simulink subsystem "switch_states"  (R2024a)
settings: Solver=VariableStepAuto  StartTime=0.0  StopTime=10.0  RelTol=1e-3
settings Model: Creator=javeed  LastModifiedBy=javeed

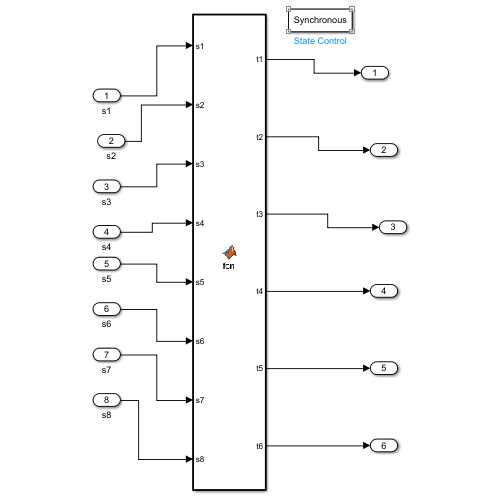
[thumbnail: Simulink's stored preview of the top-level diagram]
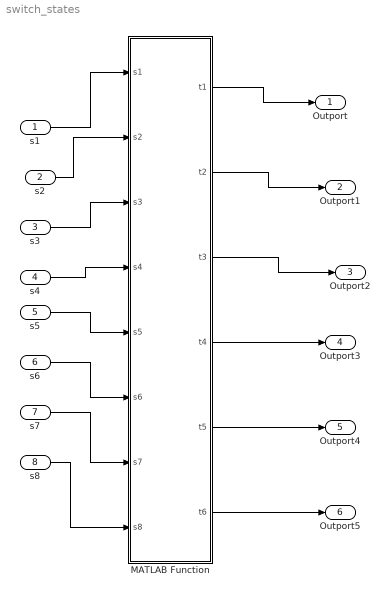
== system switch_states ==
  s1 : Inport
  s2 : Inport  Port=2
  s3 : Inport  Port=3
  s4 : Inport  Port=4
  s5 : Inport  Port=5
  s6 : Inport  Port=6
  s7 : Inport  Port=7
  s8 : Inport  Port=8
  MATLAB Function : MATLAB Function  TreatAsAtomicUnit=on
  Outport : Outport
  Outport1 : Outport  Port=2
  Outport2 : Outport  Port=3
  Outport3 : Outport  Port=4
  Outport4 : Outport  Port=5
  Outport5 : Outport  Port=6
  wires:
  s1/1 -> MATLAB Function/1(s1)
  s2/1 -> MATLAB Function/2(s2)
  s3/1 -> MATLAB Function/3(s3)
  s4/1 -> MATLAB Function/4(s4)
  s5/1 -> MATLAB Function/5(s5)
  s6/1 -> MATLAB Function/6(s6)
  s7/1 -> MATLAB Function/7(s7)
  s8/1 -> MATLAB Function/8(s8)
  MATLAB Function/1(t1) -> Outport/1
  MATLAB Function/2(t2) -> Outport1/1
  MATLAB Function/3(t3) -> Outport2/1
  MATLAB Function/4(t4) -> Outport3/1
  MATLAB Function/5(t5) -> Outport4/1
  MATLAB Function/6(t6) -> Outport5/1

== matlab function switch_states/MATLAB Function ==
  data: s1 input boolean; t1 output; s2 input; s3 input; s4 input; s5 input; s6 input; s7 input; s8 input; t2 output; t3 output; t4 output; t5 output; t6 output
function [t1,t2,t3,t4,t5,t6] = fcn(s1,s2,s3,s4,s5,s6,s7,s8)
    % Define the state matrix from the inputs
    state_mat = [s1,s2,s3,s4,s5,s6,s7,s8];
    
    % Define the switching table
    switching_table = [
        1 0 1 0 1 0;
        1 0 0 0 1 1;
        0 0 1 1 1 0;
        0 0 0 1 1 1;
        1 1 1 0 0 0;
        1 1 0 0 0 1;
        0 1 1 1 0 0;
        0 1 0 1 0 1;
    ];
    switching_table = logical(switching_table);
    % Define a mapping from state_mat to row indices in the switching table
    state_map = [
        [1 0 0 0 0 0 0 0]; % state 1
        [0 1 0 0 0 0 0 0]; % state 2
        [0 0 1 0 0 0 0 0]; % state 3
        [0 0 0 1 0 0 0 0]; % state 4
        [0 0 0 0 1 0 0 0]; % state 5
        [0 0 0 0 0 1 0 0]; % state 6
        [0 0 0 0 0 0 1 0]; % state 7
        [0 0 0 0 0 0 0 1]; % state 8
    ];
    
    % Initialize output variables
    t1 = false;
    t2 = false;
    t3 = false;
    t4 = false;
    t5 = false;
    t6 = false;
    
    % Loop through the state_map to find the correct state index
    for i = 1:size(state_map, 1)
        if isequal(state_mat, state_map(i,:))
            % Get the row from the switching_table based on the state index
            row = switching_table(i, :);
            % Assign the values to the output variables
            [t1, t2, t3, t4, t5, t6] = deal(row(1), row(2), row(3), row(4), row(5), row(6));
            return;
        end
    end
end
